simulink model "prob1"  (R2020b)
settings: Solver=VariableStepAuto  StartTime=0.0  StopTime=10.0  RelTol=1e-3
values from neighbouring files (symbols this model uses):
  b = 50    [variables_value.mat]
  k1 = 50    [variables_value.mat]
  M1 = 100    [variables_value.mat]
undefined symbols (not defined in the file or in its folder): k12, M2
settings Model: Creator=DELL  LastModifiedBy=DELL

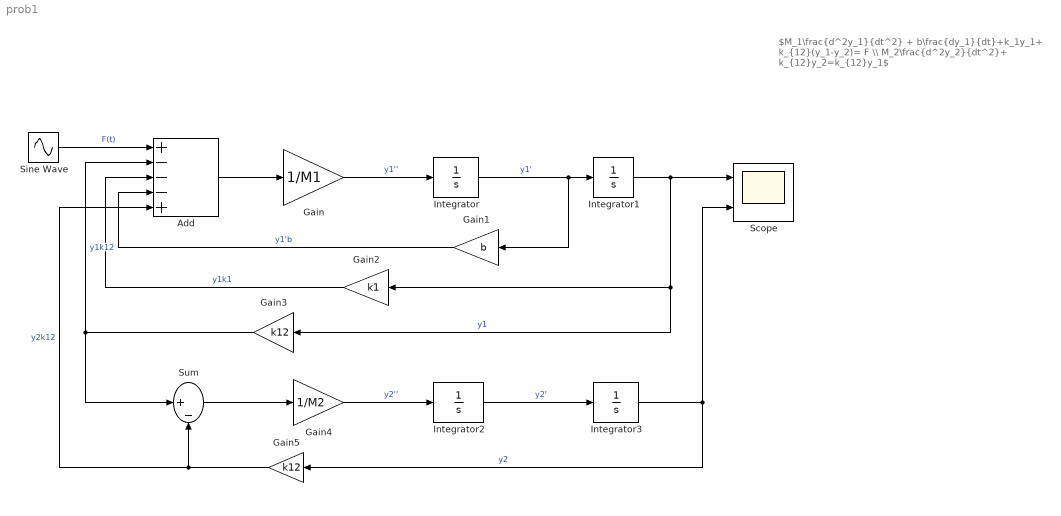
== system prob1 ==
  note: $M_1\frac{d^2y_1}{dt^2} + b\frac{dy_1}{dt}+k_1y_1+ k_{12}(y_1-y_2)= F \\ M_2\frac{d^2y_2}{dt^2}+ k_{12}y_2=k_{12}y_1$
  Add : Sum  Inputs=+---+
  Gain : Gain  Gain=1/M1
  Gain1 : Gain  Gain=b
  Gain2 : Gain  Gain=k1
  Gain3 : Gain  Gain=k12
  Gain4 : Gain  Gain=1/M2
  Gain5 : Gain  Gain=k12
  Integrator{,1..3} (4 alike) : Integrator
  Scope : Scope  NumInputPorts=2
  Sine Wave : Sin  Amplitude=2  Frequency=10  SampleTime=0
  Sum : Sum  Inputs=|+-
  wires:
  Integrator/1 -> Gain1/1, Integrator1/1  "y1'"
  Gain/1 -> Integrator/1  "y1''"
  Add/1 -> Gain/1
  Integrator1/1 -> Gain3/1, Gain2/1, Scope/1  "y1"
  Gain2/1 -> Add/3  "y1k1"
  Gain3/1 -> Add/2, Sum/1  "y1k12"
  Gain1/1 -> Add/4  "y1'b"
  Sum/1 -> Gain4/1
  Integrator2/1 -> Integrator3/1  "y2'"
  Gain4/1 -> Integrator2/1  "y2''"
  Integrator3/1 -> Gain5/1, Scope/2  "y2"
  Gain5/1 -> Sum/2, Add/5  "y2k12"
  Sine Wave/1 -> Add/1  "F(t)"
